simulink model "Part1"  (R2017b)
settings: Solver=FixedStepAuto  StartTime=0.0  StopTime=inf  RelTol=1e-3  EnableMultiTasking=on
undefined symbols (not defined in the file): D10, D11, D12, D2, D4, D5, D7, D8, D9, PTA0, PTA2, PTB23, PTB9, PTC3, PTC4, PTD0, PTD2, PTD3
libraries: frdmk64flib x9
settings Model: ExtModeTrigDuration=5  Creator=bajwam1  LastModifiedBy=muralitm
settings OptimizationCC: PassReuseOutputArgsAs=Individual arguments  MaxStackSize=64
settings DebuggingCC: ParameterTunabilityLossMsg=error
settings HardwareCC: ProdBitPerPointer=32  ProdBitPerSizeT=32  ProdBitPerPtrDiffT=32  ProdLargestAtomicInteger=Long  ProdLargestAtomicFloat=Double  ProdWordSize=32  ProdHWDeviceType=ARM Compatible->ARM Cortex
settings SFSimCC: MATLABDynamicMemAlloc=off
settings RTWCC: SystemTargetFile=ert.tlc  HardwareBoard=NXP FRDM-K64F  TemplateMakefile=ert_default_tmf  GenerateReport=on  Toolchain=GNU Tools for ARM Embedded Processors  IncludeHyperlinkInReport=on  LaunchReport=on  GenerateTraceInfo=on  GenerateTraceReport=on  GenerateTraceReportSl=on  GenerateTraceReportSf=on  GenerateTraceReportEml=on
settings CodeAppCC: ForceParamTrailComments=on  IgnoreCustomStorageClasses=off  OperatorAnnotations=on  SimulinkDataObjDesc=on  SFDataObjDesc=on  InsertBlockDesc=on

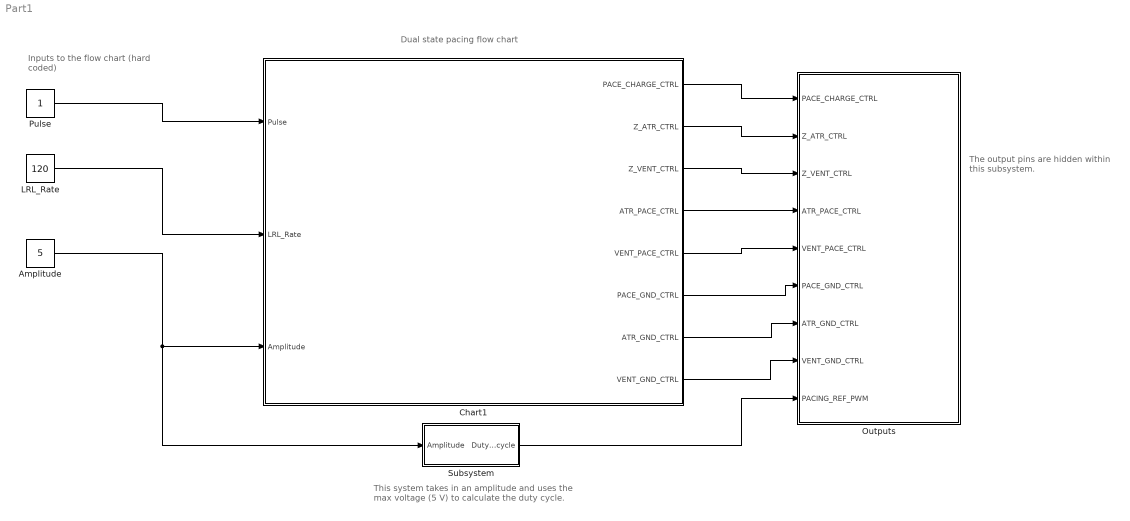
== system Part1 ==
  note: Inputs to the flow chart
      | (hard coded)
  note: Dual state pacing flow chart
  note: The output pins are hidden within
      | this subsystem.
  note: This system takes in an amplitude and uses the
      | max voltage (5 V) to calculate the duty cycle.
  "Amplitude " : Constant  Value=5
  Chart1 : Stateflow chart  TreatAsAtomicUnit=on
  LRL_Rate : Constant  Value=120
  Outputs : Subsystem
  Pulse : Constant
  Subsystem : Subsystem
  wires:
  Chart1/5(VENT_PACE_CTRL) -> Outputs/5(VENT_PACE_CTRL)
  Chart1/8(VENT_GND_CTRL) -> Outputs/8(VENT_GND_CTRL)
  Chart1/4(ATR_PACE_CTRL) -> Outputs/4(ATR_PACE_CTRL)
  Chart1/2(Z_ATR_CTRL) -> Outputs/2(Z_ATR_CTRL)
  Chart1/6(PACE_GND_CTRL) -> Outputs/6(PACE_GND_CTRL)
  Chart1/3(Z_VENT_CTRL) -> Outputs/3(Z_VENT_CTRL)
  Chart1/7(ATR_GND_CTRL) -> Outputs/7(ATR_GND_CTRL)
  LRL_Rate/1 -> Chart1/2(LRL_Rate)
  "Amplitude "/1 -> Subsystem/1(Amplitude), Chart1/3(Amplitude)
  Chart1/1(PACE_CHARGE_CTRL) -> Outputs/1(PACE_CHARGE_CTRL)
  Pulse/1 -> Chart1/1(Pulse)
  Subsystem/1(Duty_cycle) -> Outputs/9(PACING_REF_PWM)

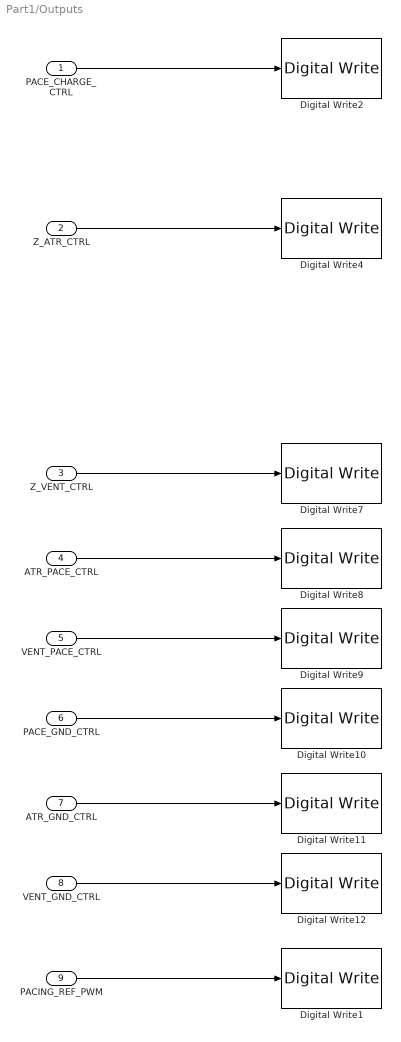
== system Part1/Outputs ==
  PACE_CHARGE_CTRL : Inport
  Z_ATR_CTRL : Inport  Port=2
  Z_VENT_CTRL : Inport  Port=3
  ATR_PACE_CTRL : Inport  Port=4
  VENT_PACE_CTRL : Inport  Port=5
  PACE_GND_CTRL : Inport  Port=6
  ATR_GND_CTRL : Inport  Port=7
  VENT_GND_CTRL : Inport  Port=8
  PACING_REF_PWM : Inport  Port=9
  Digital Write1 : frdmk64flib/Digital Write  Whichpin=PTA2 (D5)
      settings: SourceProductName=Simulink Coder Support Package for NXP FRDM-K64F Board
  Digital Write10 : frdmk64flib/Digital Write  Whichpin=PTD0 (D10)
      settings: SourceProductName=Simulink Coder Support Package for NXP FRDM-K64F Board
  Digital Write11 : frdmk64flib/Digital Write  Whichpin=PTD2 (D11)
      settings: SourceProductName=Simulink Coder Support Package for NXP FRDM-K64F Board
  Digital Write12 : frdmk64flib/Digital Write  Whichpin=PTD3 (D12)
      settings: SourceProductName=Simulink Coder Support Package for NXP FRDM-K64F Board
  Digital Write2 : frdmk64flib/Digital Write  Whichpin=PTB9 (D2)
      settings: SourceProductName=Simulink Coder Support Package for NXP FRDM-K64F Board
  Digital Write4 : frdmk64flib/Digital Write  Whichpin=PTB23 (D4)
      settings: SourceProductName=Simulink Coder Support Package for NXP FRDM-K64F Board
  Digital Write7 : frdmk64flib/Digital Write  Whichpin=PTC3 (D7)
      settings: SourceProductName=Simulink Coder Support Package for NXP FRDM-K64F Board
  Digital Write8 : frdmk64flib/Digital Write  Whichpin=PTA0 (D8)
      settings: SourceProductName=Simulink Coder Support Package for NXP FRDM-K64F Board
  Digital Write9 : frdmk64flib/Digital Write  Whichpin=PTC4 (D9)
      settings: SourceProductName=Simulink Coder Support Package for NXP FRDM-K64F Board
  wires:
  PACE_CHARGE_CTRL/1 -> Digital Write2/1
  Z_ATR_CTRL/1 -> Digital Write4/1
  Z_VENT_CTRL/1 -> Digital Write7/1
  ATR_PACE_CTRL/1 -> Digital Write8/1
  VENT_PACE_CTRL/1 -> Digital Write9/1
  PACE_GND_CTRL/1 -> Digital Write10/1
  ATR_GND_CTRL/1 -> Digital Write11/1
  VENT_GND_CTRL/1 -> Digital Write12/1
  PACING_REF_PWM/1 -> Digital Write1/1

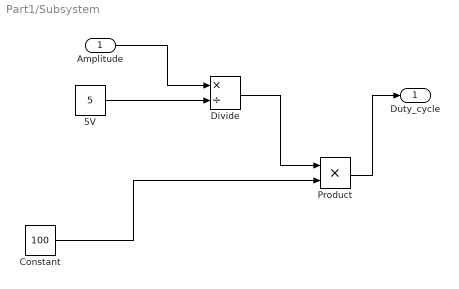
== system Part1/Subsystem ==
  Amplitude : Inport
  5V : Constant  Value=5
  Constant : Constant  Value=100
  Divide : Product  Inputs=*/
  Product : Product
  Duty_cycle : Outport  OutMin=0  OutMax=100
  wires:
  Amplitude/1 -> Divide/1
  Constant/1 -> Product/2
  Divide/1 -> Product/1
  Product/1 -> Duty_cycle/1
  5V/1 -> Divide/2

== stateflow chart Part1/Chart1 ==
  state CHARGING
    entry:
    ATR_PACE_CTRL = false
    VENT_PACE_CTRL =true
    PACE_CHARGE_CTRL = true
    PACE_GND_CTRL = true
    Z_ATR_CTRL = false
    Z_VENT_CTRL = false
    ATR_GND_CTRL = false
    VENT_GND_CTRL = false
  state PACING
    entry:
    PACE_CHARGE_CTRL = false
    PACE_GND_CTRL = true
    ATR_PACE_CTRL = false
    ATR_GND_CTRL = false
    Z_ATR_CTRL = false
    Z_VENT_CTRL = false
    VENT_GND_CTRL = true
    VENT_PACE_CTRL = false
  note: Pace Ready
  note: Recharge Ready
  note: This is the pacing state that discharges
      | the capacitor (C22) into the ventricle and
      | charges the capacitor (C21).
  note: This charging state charges the capacitor
      | C22 and discharges the blocking capacitor.
  (default) -> CHARGING
  CHARGING -> PACING : after(Pulse, msec)
  PACING -> CHARGING : after((LRL_Rate-Pulse), msec)
  data: PACE_CHARGE_CTRL output boolean; Z_ATR_CTRL output boolean; Z_VENT_CTRL output boolean; ATR_PACE_CTRL output boolean; VENT_PACE_CTRL output boolean; PACE_GND_CTRL output boolean; ATR_GND_CTRL output boolean; VENT_GND_CTRL output boolean; Pulse input; LRL_Rate input; Amplitude input
